simulink model "PROPELLER_BEM_SIMULINK"  (R2018a)
settings: Solver=VariableStepAuto  StartTime=0.0  StopTime=100  RelTol=1e-3
libraries: simulink x2
settings Model: Creator=SAMSUNG  LastModifiedBy=Usuario

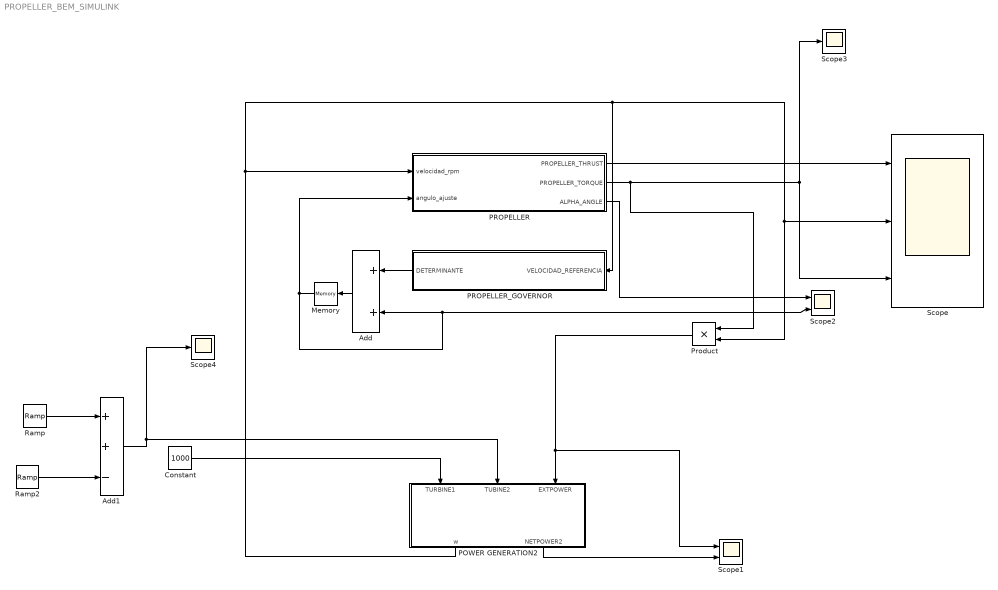
== system PROPELLER_BEM_SIMULINK ==
  Add : Sum
  Add1 : Sum  Inputs=++-
  Constant : Constant  Value=1000
  Memory : Memory
  POWER GENERATION2 : Subsystem
  PROPELLER : MATLAB Function  TreatAsAtomicUnit=on
  PROPELLER_GOVERNOR : MATLAB Function  TreatAsAtomicUnit=on
  Product : Product
  Ramp : simulink/Sources/Ramp  slope=4500  start=10  InitialOutput=5000
  Ramp2 : simulink/Sources/Ramp  slope=4500  start=20  InitialOutput=0
  Scope : Scope  NumInputPorts=3
  Scope1 : Scope  NumInputPorts=2
  Scope2 : Scope  NumInputPorts=2
  Scope3 : Scope
  Scope4 : Scope
  wires:
  Constant/1 -> POWER GENERATION2/1(TURBINE1)
  Product/1 -> Scope1/1, POWER GENERATION2/3(EXTPOWER)
  PROPELLER/2(PROPELLER_TORQUE) -> Product/1, Scope3/1, Scope/3
  POWER GENERATION2/2(NETPOWER2) -> Scope1/2
  Memory/1 -> Scope2/2, Add/2, PROPELLER/2(angulo_ajuste)
  POWER GENERATION2/1(w) -> PROPELLER_GOVERNOR/1(VELOCIDAD_REFERENCIA), Product/2, Scope/2, PROPELLER/1(velocidad_rpm)
  Add/1 -> Memory/1
  PROPELLER_GOVERNOR/1(DETERMINANTE) -> Add/1
  PROPELLER/3(ALPHA_ANGLE) -> Scope2/1
  PROPELLER/1(PROPELLER_THRUST) -> Scope/1
  Ramp/1 -> Add1/1
  Ramp2/1 -> Add1/3
  Add1/1 -> POWER GENERATION2/2(TUBINE2), Scope4/1

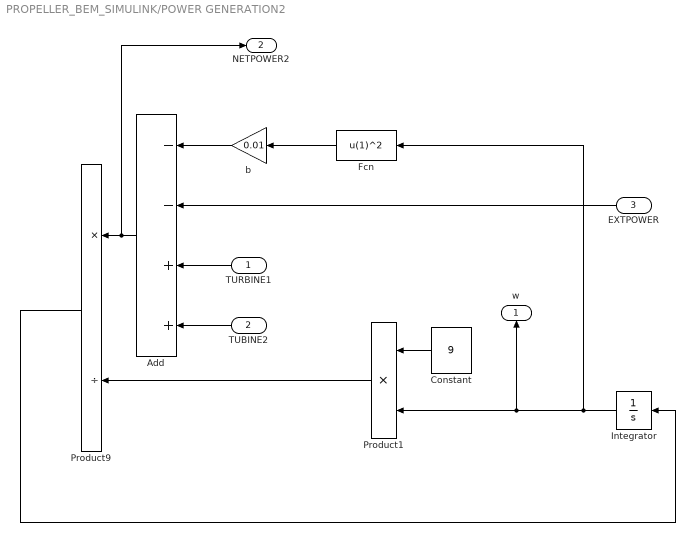
== system PROPELLER_BEM_SIMULINK/POWER GENERATION2 ==
  TURBINE1 : Inport
  TUBINE2 : Inport  Port=2
  EXTPOWER : Inport  Port=3
  Add : Sum  Inputs=--++
  Constant : Constant  Value=9
  Fcn : Fcn  Expr=u(1)^2
  Integrator : Integrator  InitialCondition=90
  Product1 : Product
  Product9 : Product  Inputs=*/
  b : Gain  Gain=0.01
  w : Outport
  NETPOWER2 : Outport  Port=2
  wires:
  Product1/1 -> Product9/2
  Add/1 -> NETPOWER2/1, Product9/1
  Product9/1 -> Integrator/1
  TUBINE2/1 -> Add/4
  TURBINE1/1 -> Add/3
  Constant/1 -> Product1/1
  Integrator/1 -> Fcn/1, Product1/2, w/1
  Fcn/1 -> b/1
  b/1 -> Add/1
  EXTPOWER/1 -> Add/2

== matlab function PROPELLER_BEM_SIMULINK/PROPELLER ==
  data: velocidad_rpm input; PROPELLER_THRUST output; angulo_ajuste input; PROPELLER_TORQUE output; ALPHA_ANGLE output
function  [PROPELLER_THRUST,PROPELLER_TORQUE,ALPHA_ANGLE]= fcn(velocidad_rpm,angulo_ajuste)
 ...........................PARAMETROS INICIALES ...........................
numero_de_palas=4;                  %NUMERO DE PALAS QUE TIENE EL PROPELLER
radio_maxima_pala=0.9;              %RADIO MAXIMO DE LA PALA DEL PROPELLER
radio_base_pala=0.2;                %RADIO EN LA BASE DE LA PALA DEL PROPELLER
theta_inicial=10+angulo_ajuste;                   %ANGULO GEOMETRICO DEL PROPELLER EN LA BASE
theta_final=20+angulo_ajuste;                     %ANGULO GEOMETRICO EN LA BASE DEL PROPELLER
numero_de_divisiones=10;            %DIVISIONES QUE SE ESTIMAN PARA LA PALA 
velocidad_inf=13;                   %VELOCIDAD DEL AIRE ANTES DE ENTRAR AL PROPELLER
b1=0.15;                             %ANGULAR INFLOW FACTOR (SWIRL FACTOR) (INITIAL)
a1=4;                             %AXIAL INFLOW FACTOR  (INITIAL)
densidad_aire=1.222;                %DENSIDAD AIRE EN KG/M^3
CL=0.6;
CD=0.1;
C_base=0.12 ;                          %Chord en la base de la paleta
C_punta=0.08;                           %Chord en la punta de la paleta
W=1.5;                              %METODO DE RELAJACION 0<W<2 
ERROR=0.002;
numero_maximo_iteraciones=1200;  

STEP_pala=(radio_maxima_pala-radio_base_pala)/numero_de_divisiones ;%STEP DEL RADIO
STEP_theta=(theta_final-theta_inicial)/(numero_de_divisiones-1) ;%STEP DEL ANGULO 
STEP_Chord=(C_base-C_punta)/(numero_de_divisiones-1);
PALA=[radio_base_pala:STEP_pala:radio_maxima_pala]' ; % DIVISION DE LAS PALAS
tip_pala_por_divisiones = PALA(2:11,1);
THETA=[theta_inicial:STEP_theta:theta_final]'*pi/180;  %DIVISION DE ANGULO
CHORD=[C_punta:STEP_Chord:C_base]';
velocidad_radianes=velocidad_rpm;
velocidad_punta_pala=tip_pala_por_divisiones(:,1)*velocidad_radianes; % VELOCIDAD DE LA PUNTA DE LA PALA
a=zeros(numero_de_divisiones,1)+a1;
b=zeros(numero_de_divisiones,1)+b1; 
%....................CALCULO DE VELOCIDAD RELATIVA ........................



V1=zeros(max(size(velocidad_punta_pala)),1);   % VELOCIDAD RELATIVA DEL AIRE sqrt(V2^2+V1^2)
V0=zeros(max(size(velocidad_punta_pala)),1);
V2=zeros(max(size(velocidad_punta_pala)),1);
ALPHA= zeros(max(size(velocidad_punta_pala)),1);
EMPUJE=zeros(max(size(velocidad_punta_pala)),1);
numero_puntos_a_bajo_pararametro_error=0;
numero_puntos_b_bajo_pararametro_error=0;
numero_iteraciones_alcanzadas=0;
DQDR=zeros(max(size(velocidad_punta_pala)),1);
DTDR=zeros(max(size(velocidad_punta_pala)),1);
for k=1:numero_maximo_iteraciones

a_anterior=a;
b_anterior=b;
V0=velocidad_inf*(1+a);                                      % VELOCIDAD AXIAL AL ENTRAR AL PROPELLER
V2=velocidad_punta_pala.*(1-b);                             % VELOCIADAD DEL AIRE EN LA PUNTA DEL CADA ELEMENTO

for i=1:max(size(V2 ))
 
    V1(i,1)=sqrt(V2(i ,1).*V2(i ,1)+V0(i,1).*V0(i,1) )
  
    ALPHA(i,1)=THETA(i,1)-atan(V0(i,1)./V2(i,1));
    DTDR(i,1)=(1/2)*densidad_aire.*V1(i,1).*V1(i,1).*CHORD(i,1).*(CL.*cos(ALPHA(i,1))-CD.*sin(ALPHA(i,1))).*numero_de_palas;
    DQDR(i,1)=(1/2)*densidad_aire*V1(i,1).*V1(i,1)*CHORD(i,1)*tip_pala_por_divisiones(i,1).*(CL*sin(ALPHA(i,1))+CD*cos(ALPHA(i,1)))*numero_de_palas;
    k=4*densidad_aire*pi*tip_pala_por_divisiones(i,1)*velocidad_inf*velocidad_inf;
    a(i,1)=W*(-k+sqrt(k*k+4*k*DTDR(i,1)))./(2*k)+(1-W).*a(i,1);
    b(i,1)= W*(DQDR(i,1)./(4*densidad_aire*pi*tip_pala_por_divisiones(i,1)*tip_pala_por_divisiones(i,1)*tip_pala_por_divisiones(i,1)*velocidad_inf*velocidad_inf*velocidad_radianes*(a(i,1)+1)))+(1-W)*b(i,1);   
end
R_a=0;
R_b=0;
break_loop_a=0;
break_loop_b=0;

for k=1:max(size(V2(:,1)))
if abs((a(k,1)-a_anterior(k,1)))<ERROR
    R_a=R_a+1;
    if R_a==max(size(V2(:,1)))
        numero_puntos_a_bajo_pararametro_error=R_a;
        break_loop_a=1;
    end
end
numero_puntos_a_bajo_pararametro_error=R_a;
end


for k=1:max(size(V2(:,1)))
if abs((b(k,1)-b_anterior(k,1)))<ERROR
    R_b=R_b+1;
    if R_b==max(size(V2(:,1)))
        numero_puntos_b_bajo_pararametro_error=R_b;
        break_loop_b=1;
    end
end
numero_puntos_b_bajo_pararametro_error=R_b;
end

numero_iteraciones_alcanzadas=numero_iteraciones_alcanzadas+1;
if  (break_loop_a)==1 && (break_loop_b)==1
    break
end
end
EMPUJE=2*pi*densidad_aire*(PALA(2:11,1).*PALA(2:11,1)-PALA(1:10,1).*PALA(1:10,1))*velocidad_inf*velocidad_inf.*(1+a(:,1)).*a(:,1);
TORQUE=pi*densidad_aire*(PALA(2:11,1).*PALA(2:11,1).*PALA(2:11,1).*PALA(2:11,1)-PALA(1:10,1).*PALA(1:10,1).*PALA(1:10,1).*PALA(1:10,1))*velocidad_inf*velocidad_inf.*(1+a(:,1)).*b*velocidad_radianes;

 
EMPUJE1=sum(EMPUJE);
TORQUE1=sum(TORQUE);
ALPHA_ANGLE=theta_inicial; 
PROPELLER_TORQUE=TORQUE1;
PROPELLER_THRUST=EMPUJE1;

== matlab function PROPELLER_BEM_SIMULINK/PROPELLER_GOVERNOR ==
  data: VELOCIDAD_REFERENCIA input; DETERMINANTE output
function DETERMINANTE= fcn(VELOCIDAD_REFERENCIA)

DETERMINANTE1=0;
if VELOCIDAD_REFERENCIA<198
    DETERMINANTE1=-1;
end
if VELOCIDAD_REFERENCIA>209
    DETERMINANTE1=1;
end
     
DETERMINANTE= DETERMINANTE1;
